simulink model "tether000Test1"  (R2018b)
settings: Solver=VariableStepAuto  StartTime=0.0  StopTime=duration_s  FixedStep=.1  RelTol=1e-3
values from neighbouring files (symbols this model uses):
  constantVelocity = 1    [tether000Test_ts.m]
  positionTopNode = thr.tether1.initAirNodePos.Value*ones(1,simDuration)    [tether000Test_ts.m]
  simDuration = 20    [tether000Test_ts.m]    (also in tether000_tsmc.m = 100)
  tetherLength = totalUnstchLength    (= 200)    [tether000Test_ts.m]
  thr = OCT.tethers    [tether000Test_ts.m]    (also in tether000_tsmc.m)
  velocityTopNode = [1;1;1]*zeros(1,simDuration)    [tether000Test_ts.m]
libraries: vectorNormalizer_ul x1, tethers_cl x1
settings Model: Creator=James Reed  LastModifiedBy=James Reed

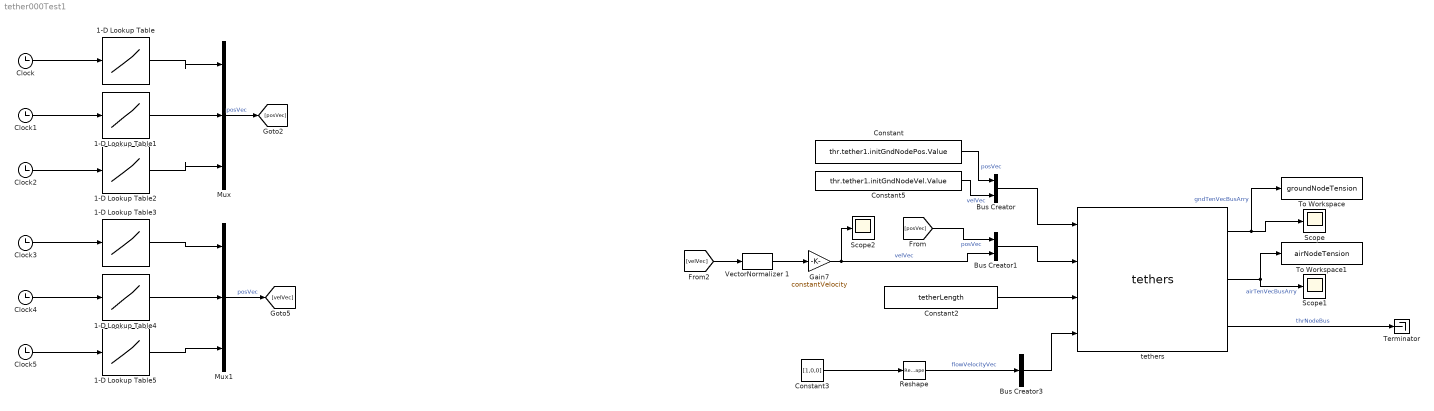
== system tether000Test1 ==
  1-D Lookup Table : Lookup_n-D  NumberOfTableDimensions=1  BreakpointsForDimension1=1:simDuration  Table=positionTopNode(1,:)  InternalRulePriority=Speed  RndMeth=Simplest  InputSameDT=on
  1-D Lookup Table1 : Lookup_n-D  NumberOfTableDimensions=1  BreakpointsForDimension1=1:simDuration  Table=positionTopNode(2,:)  InterpMethod=Linear Lagrange  InternalRulePriority=Speed  RndMeth=Simplest  InputSameDT=on
  1-D Lookup Table2 : Lookup_n-D  NumberOfTableDimensions=1  BreakpointsForDimension1=1:simDuration  Table=positionTopNode(3,:)  InterpMethod=Linear Lagrange  InternalRulePriority=Speed  RndMeth=Simplest  InputSameDT=on
  1-D Lookup Table3 : Lookup_n-D  NumberOfTableDimensions=1  BreakpointsForDimension1=1:simDuration  Table=velocityTopNode(1,:)  InterpMethod=Linear Lagrange  InternalRulePriority=Speed  RndMeth=Simplest  InputSameDT=on
  1-D Lookup Table4 : Lookup_n-D  NumberOfTableDimensions=1  BreakpointsForDimension1=1:simDuration  Table=velocityTopNode(2,:)  InternalRulePriority=Speed  RndMeth=Simplest  InputSameDT=on
  1-D Lookup Table5 : Lookup_n-D  NumberOfTableDimensions=1  BreakpointsForDimension1=1:simDuration  Table=velocityTopNode(3,:)  InterpMethod=Linear Lagrange  InternalRulePriority=Speed  RndMeth=Simplest  InputSameDT=on
  Bus Creator : BusCreator  Inputs=2  OutDataTypeStr=Bus: thrAttachPtKinematicsBus  NonVirtualBus=on
  Bus Creator1 : BusCreator  Inputs=2  OutDataTypeStr=Bus: thrAttachPtKinematicsBus  NonVirtualBus=on
  Bus Creator3 : BusCreator  Inputs=1  OutDataTypeStr=Bus:envBus
  Clock{,1..5} (6 alike) : Clock
  Constant : Constant  Value=thr.tether1.initGndNodePos.Value
  Constant2 : Constant  Value=tetherLength
  Constant3 : Constant  Value=[1,0,0]
  Constant5 : Constant  Value=thr.tether1.initGndNodeVel.Value
  Gain7 : Gain  Gain=constantVelocity
  Mux : Mux  Inputs=3
  Mux1 : Mux  Inputs=3
  Reshape : Reshape  OutputDimensionality=Column vector (2-D)
  Scope : Scope
  Scope1 : Scope
  Scope2 : Scope
  Terminator : Terminator
  To Workspace : ToWorkspace  VariableName=groundNodeTension  SaveFormat=Timeseries  SampleTime=-1
  To Workspace1 : ToWorkspace  VariableName=airNodeTension  SaveFormat=Timeseries  SampleTime=-1
  VectorNormalizer 1 : vectorNormalizer_ul/VectorNormalizer   SystemSampleTime=-1
  tethers : tethers_cl/tethers  SystemSampleTime=-1
      link override tether000: thrStructure=thr.struct('OCT.tether')
  wires:
  tethers/3 -> Terminator/1  "thrNodeBus"
  Constant2/1 -> tethers/3
  tethers/2 -> To Workspace1/1, Scope1/1  "airTenVecBusArry"
  tethers/1 -> To Workspace/1, Scope/1  "gndTenVecBusArry"
  Constant/1 -> Bus Creator/1  "posVec"
  Constant5/1 -> Bus Creator/2  "velVec"
  Bus Creator/1 -> tethers/1
  Bus Creator1/1 -> tethers/2
  Gain7/1 -> Bus Creator1/2, Scope2/1  "velVec"
  Constant3/1 -> Reshape/1
  Bus Creator3/1 -> tethers/4
  Reshape/1 -> Bus Creator3/1  "flowVelocityVec"
  1-D Lookup Table1/1 -> Mux/2
  1-D Lookup Table/1 -> Mux/1
  1-D Lookup Table2/1 -> Mux/3
  Mux/1 -> [posVec]  "posVec"
  [posVec] -> Bus Creator1/1  "posVec"
  1-D Lookup Table5/1 -> Mux1/3
  1-D Lookup Table4/1 -> Mux1/2
  1-D Lookup Table3/1 -> Mux1/1
  Mux1/1 -> [velVec]  "posVec"
  VectorNormalizer 1/1 -> Gain7/1
  [velVec] -> VectorNormalizer 1/1
  Clock/1 -> 1-D Lookup Table/1
  Clock1/1 -> 1-D Lookup Table1/1
  Clock2/1 -> 1-D Lookup Table2/1
  Clock3/1 -> 1-D Lookup Table3/1
  Clock4/1 -> 1-D Lookup Table4/1
  Clock5/1 -> 1-D Lookup Table5/1
